simulink model "simulation"  (R2021a)
settings: Solver=VariableStepAuto  StartTime=0.0  StopTime=50.0  FixedStep=0.00009  RelTol=1e-3
values from neighbouring files (symbols this model uses):
  a21 = -2*(k+K)/(2*Mt+9*m)    (= -2436.05359318)    [parameters_initialization.m]
  a22 = -2*(b+Bp)/(2*Mt+9*m)    (= -0.219244823386)    [parameters_initialization.m]
  a23 = 2*Ap/(2*Mt+9*m)    (= 1.70523751523e-05)    [parameters_initialization.m]
  a24 = 2*k/(2*Mt+9*m)    (= 2436.05359318)    [parameters_initialization.m]
  a25 = 2*b/(2*Mt+9*m)    (= 0.182704019488)    [parameters_initialization.m]
  a32 = -Ap*4*Be/Vt    (= -18200000000)    [parameters_initialization.m]
  a33 = -4*Be*(Kc+Ctp)/Vt    (= -2.73)    [parameters_initialization.m]
  a51 = k*6/(7*m)    (= 9523.80952381)    [parameters_initialization.m]
  a52 = b*6/(7*m)    (= 0.714285714286)    [parameters_initialization.m]
  a54 = -k*6/(7*m)    (= -9523.80952381)    [parameters_initialization.m]
  a55 = -b*6/(7*m)    (= -0.714285714286)    [parameters_initialization.m]
  b31 = Kq*Kt*4*Be/(Vt*R*r*Kf)    (= 176800000)    [parameters_initialization.m]
  h51 = (6/7)*g    (= 8.40857142857)    [parameters_initialization.m]
settings Model: Creator=st190427d  LastModifiedBy=st190427d
settings SolverCC: ZeroCrossAlgorithm=Adaptive  AlgebraicLoopSolver=TrustRegion
settings DataIOCC: ReturnWorkspaceOutputs=off
settings DebuggingCC: MaxConsecutiveZCsMsg=none  SFMachineParentedDataDiag=warning  ArithmeticOperatorsInVariantConditions=warning
settings SFSimCC: SimUseLocalCustomCode=off  CustomCodeUndefinedFunction=UseInterfaceOnly
settings RTWCC: RTWUseLocalCustomCode=off

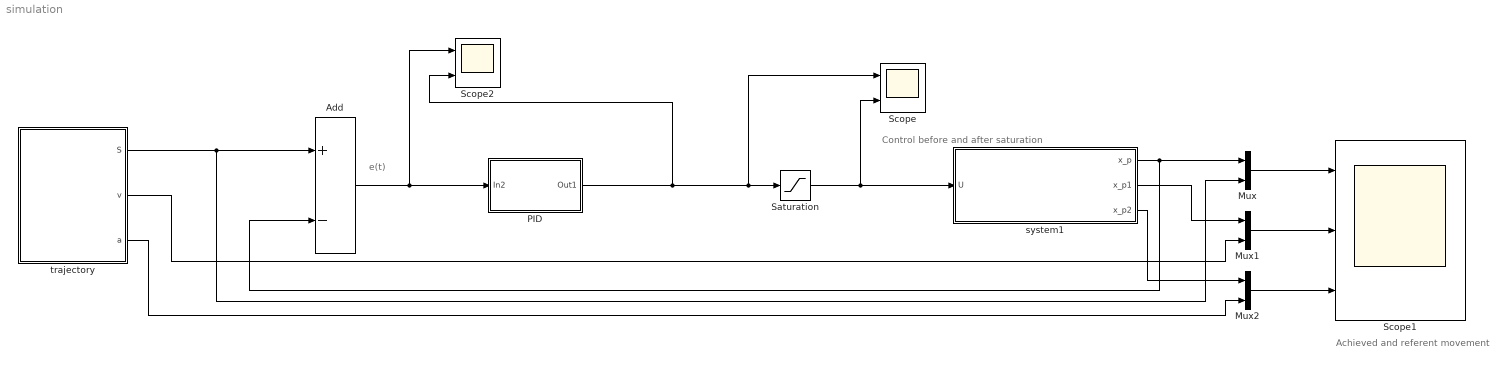
== system simulation ==
  note: e(t)
  note: Achieved and referent movement
  note: Control before and after saturation
  Add : Sum  Inputs=+-
  Mux : Mux  Inputs=2
  Mux1 : Mux  Inputs=2
  Mux2 : Mux  Inputs=2
  PID : Subsystem
  Saturation : Saturate  UpperLimit=24  LowerLimit=-24
  Scope : Scope  NumInputPorts=2
  Scope1 : Scope  NumInputPorts=3
  Scope2 : Scope  NumInputPorts=2
  system1 : Subsystem
  trajectory : Subsystem
  wires:
  trajectory/1(S) -> Mux/2, Add/1
  system1/1(x_p) -> Add/2, Mux/1
  Add/1 -> Scope2/1, PID/1(In2)
  Mux/1 -> Scope1/1
  PID/1(Out1) -> Scope2/2, Saturation/1, Scope/1
  Saturation/1 -> system1/1(U), Scope/2
  system1/2(x_p1) -> Mux1/1
  trajectory/2(v) -> Mux1/2
  system1/3(x_p2) -> Mux2/1
  trajectory/3(a) -> Mux2/2
  Mux1/1 -> Scope1/2
  Mux2/1 -> Scope1/3

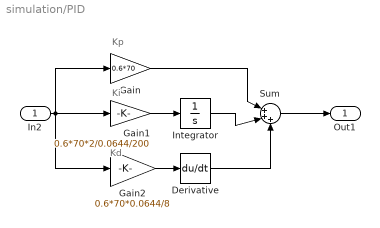
== system simulation/PID ==
  note: Kd
  note: Kp
  note: Ki
  In2 : Inport
  Derivative : Derivative
  Gain : Gain  Gain=0.6*70
  Gain1 : Gain  Gain=0.6*70*2/0.0644/200
  Gain2 : Gain  Gain=0.6*70*0.0644/8
  Integrator : Integrator
  Sum : Sum  Inputs=|+++
  Out1 : Outport  VectorParamsAs1DForOutWhenUnconnected=off
  wires:
  Gain1/1 -> Integrator/1
  In2/1 -> Gain/1, Gain2/1, Gain1/1
  Gain/1 -> Sum/1
  Sum/1 -> Out1/1
  Integrator/1 -> Sum/2
  Derivative/1 -> Sum/3
  Gain2/1 -> Derivative/1

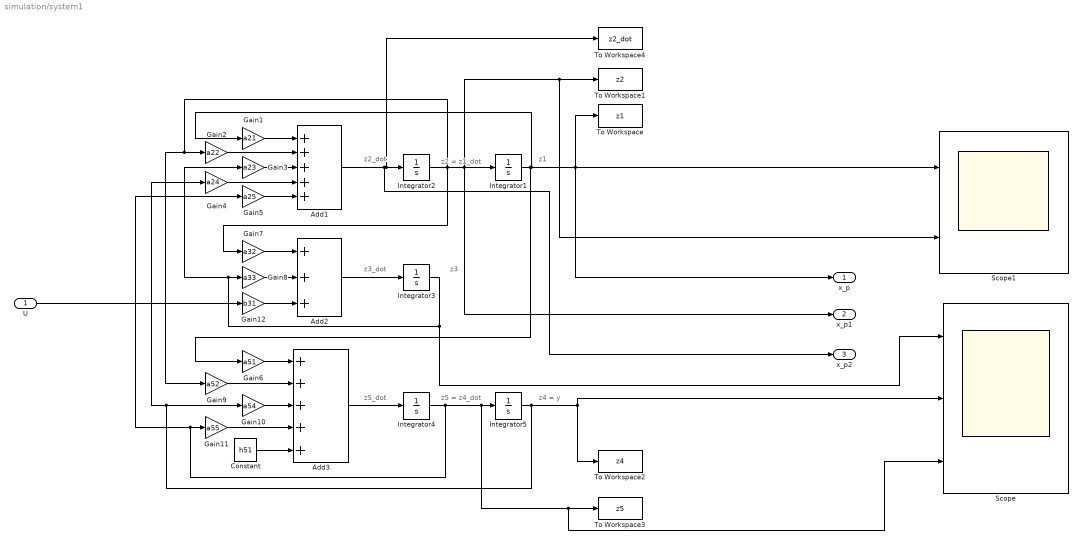
== system simulation/system1 ==
  note: z1
  note: z2 = z1_dot
  note: z2_dot
  note: z3_dot
  note: z3
  note: z4 = y
  note: z5 = z4_dot
  note: z5_dot
  U : Inport
  Add1 : Sum  Inputs=+++++
  Add2 : Sum  Inputs=+++
  Add3 : Sum  Inputs=+++++
  Constant : Constant  Value=h51
  Gain1 : Gain  Gain=a21
  Gain10 : Gain  Gain=a54
  Gain11 : Gain  Gain=a55
  Gain12 : Gain  Gain=b31
  Gain2 : Gain  Gain=a22
  Gain3 : Gain  Gain=a23
  Gain4 : Gain  Gain=a24
  Gain5 : Gain  Gain=a25
  Gain6 : Gain  Gain=a51
  Gain7 : Gain  Gain=a32
  Gain8 : Gain  Gain=a33
  Gain9 : Gain  Gain=a52
  Integrator{1..5} (5 alike) : Integrator
  Scope : Scope  NumInputPorts=3
  Scope1 : Scope  NumInputPorts=2
  To Workspace : ToWorkspace  VariableName=z1  SaveFormat=Timeseries  SampleTime=-1
  To Workspace1 : ToWorkspace  VariableName=z2  SaveFormat=Timeseries  SampleTime=-1
  To Workspace2 : ToWorkspace  VariableName=z4  SaveFormat=Timeseries  SampleTime=-1
  To Workspace3 : ToWorkspace  VariableName=z5  SaveFormat=Timeseries  SampleTime=-1
  To Workspace4 : ToWorkspace  VariableName=z2_dot  SaveFormat=Timeseries  SampleTime=-1
  x_p : Outport  VectorParamsAs1DForOutWhenUnconnected=off
  x_p1 : Outport  Port=2  VectorParamsAs1DForOutWhenUnconnected=off
  x_p2 : Outport  Port=3  VectorParamsAs1DForOutWhenUnconnected=off
  wires:
  Gain7/1 -> Add2/1
  Add1/1 -> x_p2/1, To Workspace4/1, Integrator2/1
  Gain3/1 -> Add1/3
  Add2/1 -> Integrator3/1
  Gain1/1 -> Add1/1
  Integrator1/1 -> Scope1/1, x_p/1, To Workspace/1, Gain1/1, Gain6/1
  Gain6/1 -> Add3/1
  Integrator3/1 -> Scope/1, Gain3/1, Gain8/1
  Add3/1 -> Integrator4/1
  Gain12/1 -> Add2/3
  Integrator4/1 -> Gain5/1, Gain11/1, Scope/3, To Workspace3/1, Integrator5/1
  Integrator5/1 -> To Workspace2/1, Scope/2, Gain4/1, Gain10/1
  Gain5/1 -> Add1/5
  Gain2/1 -> Add1/2
  Gain11/1 -> Add3/4
  U/1 -> Gain12/1
  Integrator2/1 -> Gain7/1, Gain9/1, Gain2/1, x_p1/1, To Workspace1/1, Scope1/2, Integrator1/1
  Gain9/1 -> Add3/2
  Gain10/1 -> Add3/3
  Gain8/1 -> Add2/2
  Gain4/1 -> Add1/4
  Constant/1 -> Add3/5

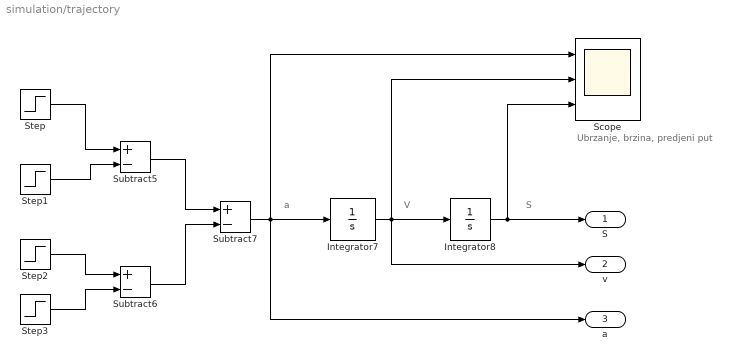
== system simulation/trajectory ==
  note: a
  note: V
  note: S
  note: Ubrzanje, brzina, predjeni put
  Integrator7 : Integrator
  Integrator8 : Integrator
  Scope : Scope  NumInputPorts=3
  Step : Step  Time=0  After=10/3  SampleTime=0
  Step1 : Step  Time=0.3  After=10/3  SampleTime=0
  Step2 : Step  Time=1.2  After=10/3  SampleTime=0
  Step3 : Step  Time=1.5  After=10/3  SampleTime=0
  Subtract5 : Sum  Inputs=+-
  Subtract6 : Sum  Inputs=+-
  Subtract7 : Sum  Inputs=+-
  S : Outport  VectorParamsAs1DForOutWhenUnconnected=off
  v : Outport  Port=2  VectorParamsAs1DForOutWhenUnconnected=off
  a : Outport  Port=3  VectorParamsAs1DForOutWhenUnconnected=off
  wires:
  Integrator8/1 -> Scope/3, S/1
  Step2/1 -> Subtract6/1
  Step1/1 -> Subtract5/2
  Subtract5/1 -> Subtract7/1
  Subtract6/1 -> Subtract7/2
  Step/1 -> Subtract5/1
  Step3/1 -> Subtract6/2
  Subtract7/1 -> a/1, Scope/1, Integrator7/1
  Integrator7/1 -> v/1, Scope/2, Integrator8/1
